simulink model "SF014A_InertiaCmpVel"  (R2013b)
settings: Solver=FixedStepDiscrete  SolverMode=SingleTasking  StartTime=0.0  StopTime=10  FixedStep=0.002  RelTol=1e-3
undefined symbols (not defined in the file): ARCHGLBPRM_2MILLISEC_SEC_F32, ARCHGLBPRM_2PI_ULS_F32, ARCHGLBPRM_PIOVER180_ULS_F32, FLTINJ_INERTIACMPVEL_INERTIACMPCMD, InertiaCmpVelDampgDecelGain, InertiaCmpVelDampgDecelGainFallSlew, InertiaCmpVelDampgGainOffThd, InertiaCmpVelDampgGainOnThd, InertiaCmpVelDecelGainEnaCal, InertiaCmpVelMotInertia, InertiaCmpVelNotchFilStruct, NOTCHFILZEROTHD_ULS_F32, SysGlbPrmSysKineRat, SysGlbPrmTorsBarStfn
libraries: FixdToFloat x13, LnrIntrpn x13, FloatToFixd x9, NxtrAbslt x4, NxtrMath x4, NxtrLim x4, simulink x2, Fil x2
(part 3 of 3)

== system SF014A_InertiaCmpVel/InertiaCmpVel/InertiaCmpVelPer1/FilterCoefCalc/Coeff_a2 ==
  FilFreqRadPs : Inport
  Constant2 : Constant  Value=ARCHGLBPRM_2MILLISEC_SEC_F32
  Constant9 : Constant  Value=2  OutDataTypeStr=single
      settings: AttributesFormatString=%<OutDataTypeStr>
  CopyRight2 : Subsystem  Description=|  mask(Copyright Information){none=on}
      | Copyright info block.                                               
      |                                                                     
      | Place copyright information at the top of every subsystem in design.
      mask prompts: none "No parameters"
      mask help: Place copyright information at the top of every subsystem in design.
      mask Display:
      | NxtrConf = 'Nexteer Confidential';
      | 
      | sys = bdroot; %handle for the current model ("system")
      | first = get_param(sys,'Created');
      | first = first(end-3:end);  %year is last four digits
      | 
      | last = get_param(sys,'LastModifiedDate');
      | if isempty(last)
      |     last = datestr(now,'yyyy');
      | else
      |     last = last(end-3:end);
      | end
      | 
      | if strcmp(first,last)
      |     fprintf('%s -- Copyright %s Nexteer',NxtrConf,first)
      | else
      |     fprintf('%s -- %s%s- %s Nexteer',NxtrConf,char(169),first,last)
      | end
  Math Function4 : Math  Operator=square  SaturateOnIntegerOverflow=on
  Product25 : Product  Inputs=**  RndMeth=Zero  OutDataTypeStr=Inherit: Same as first input
  Sum14 : Sum  OutDataTypeStr=Inherit: Same as first input
  a2 : Outport
  wires:
  FilFreqRadPs/1 -> Product25/1
  Constant2/1 -> Product25/2
  Sum14/1 -> Math Function4/1
  Math Function4/1 -> a2/1  "a2"
  Product25/1 -> Sum14/1
  Constant9/1 -> Sum14/2

== system SF014A_InertiaCmpVel/InertiaCmpVel/InertiaCmpVelPer1/FilterCoefCalc/Coeff_b0 ==
  InertiaCompCalc : Inport
  ADDCoef : Inport  Port=2
  FilFreqRadPs : Inport  Port=3
  Constant16 : Constant  Value=2  OutDataTypeStr=single
      settings: AttributesFormatString=%<OutDataTypeStr>
  Constant5 : Constant  Value=ARCHGLBPRM_2MILLISEC_SEC_F32
  Constant6 : Constant  Value=ARCHGLBPRM_2MILLISEC_SEC_F32
  CopyRight2 : Subsystem  Description=|  mask(Copyright Information){none=on}
      | Copyright info block.                                               
      |                                                                     
      | Place copyright information at the top of every subsystem in design.
      mask prompts: none "No parameters"
      mask help: Place copyright information at the top of every subsystem in design.
      mask Display:
      | NxtrConf = 'Nexteer Confidential';
      | 
      | sys = bdroot; %handle for the current model ("system")
      | first = get_param(sys,'Created');
      | first = first(end-3:end);  %year is last four digits
      | 
      | last = get_param(sys,'LastModifiedDate');
      | if isempty(last)
      |     last = datestr(now,'yyyy');
      | else
      |     last = last(end-3:end);
      | end
      | 
      | if strcmp(first,last)
      |     fprintf('%s -- Copyright %s Nexteer',NxtrConf,first)
      | else
      |     fprintf('%s -- %s%s- %s Nexteer',NxtrConf,char(169),first,last)
      | end
  Product10 : Product  Inputs=**  RndMeth=Zero  OutDataTypeStr=Inherit: Same as first input
  Product11 : Product  Inputs=**  RndMeth=Zero  OutDataTypeStr=Inherit: Same as first input
  Product23 : Product  Inputs=**  RndMeth=Zero  OutDataTypeStr=Inherit: Same as first input
  Product24 : Product  Inputs=3  RndMeth=Zero  OutDataTypeStr=Inherit: Same as first input
  Sum13 : Sum  Inputs=-+-  OutDataTypeStr=Inherit: Same as first input
  b0 : Outport
  wires:
  Constant5/1 -> Product23/1
  InertiaCompCalc/1 -> Product23/2
  Constant6/1 -> Product24/1
  FilFreqRadPs/1 -> Product24/3
  ADDCoef/1 -> Product10/1, Product24/2
  Product23/1 -> Sum13/1
  Product24/1 -> Sum13/2
  Sum13/1 -> Product11/1
  Product11/1 -> b0/1  "b0"
  Product10/1 -> Sum13/3
  Constant16/1 -> Product11/2, Product10/2

== system SF014A_InertiaCmpVel/InertiaCmpVel/InertiaCmpVelPer1/FilterCoefCalc/Coeff_b1 ==
  ADDCoef : Inport
  Constant14 : Constant  Value=2  OutDataTypeStr=single
      settings: AttributesFormatString=%<OutDataTypeStr>
  Constant17 : Constant  Value=4  OutDataTypeStr=single
      settings: AttributesFormatString=%<OutDataTypeStr>
  CopyRight2 : Subsystem  Description=|  mask(Copyright Information){none=on}
      | Copyright info block.                                               
      |                                                                     
      | Place copyright information at the top of every subsystem in design.
      mask prompts: none "No parameters"
      mask help: Place copyright information at the top of every subsystem in design.
      mask Display:
      | NxtrConf = 'Nexteer Confidential';
      | 
      | sys = bdroot; %handle for the current model ("system")
      | first = get_param(sys,'Created');
      | first = first(end-3:end);  %year is last four digits
      | 
      | last = get_param(sys,'LastModifiedDate');
      | if isempty(last)
      |     last = datestr(now,'yyyy');
      | else
      |     last = last(end-3:end);
      | end
      | 
      | if strcmp(first,last)
      |     fprintf('%s -- Copyright %s Nexteer',NxtrConf,first)
      | else
      |     fprintf('%s -- %s%s- %s Nexteer',NxtrConf,char(169),first,last)
      | end
  Product12 : Product  Inputs=**  RndMeth=Zero  OutDataTypeStr=Inherit: Same as first input
  Product8 : Product  Inputs=**  RndMeth=Zero  OutDataTypeStr=Inherit: Same as first input
  b1 : Outport
  wires:
  ADDCoef/1 -> Product8/1
  Product8/1 -> b1/1  "b1"
  Product12/1 -> Product8/2
  Constant17/1 -> Product12/1
  Constant14/1 -> Product12/2

== system SF014A_InertiaCmpVel/InertiaCmpVel/InertiaCmpVelPer1/FilterCoefCalc/Coeff_b2 ==
  InertiaCompCalc : Inport
  " FilFreqRadPs" : Inport  Port=2
  ADDCoef : Inport  Port=3
  Constant1 : Constant  Value=ARCHGLBPRM_2MILLISEC_SEC_F32
  Constant11 : Constant  Value=2  OutDataTypeStr=single
      settings: AttributesFormatString=%<OutDataTypeStr>
  Constant13 : Constant  Value=2  OutDataTypeStr=single
      settings: AttributesFormatString=%<OutDataTypeStr>
  Constant3 : Constant  Value=ARCHGLBPRM_2MILLISEC_SEC_F32
  CopyRight2 : Subsystem  Description=|  mask(Copyright Information){none=on}
      | Copyright info block.                                               
      |                                                                     
      | Place copyright information at the top of every subsystem in design.
      mask prompts: none "No parameters"
      mask help: Place copyright information at the top of every subsystem in design.
      mask Display:
      | NxtrConf = 'Nexteer Confidential';
      | 
      | sys = bdroot; %handle for the current model ("system")
      | first = get_param(sys,'Created');
      | first = first(end-3:end);  %year is last four digits
      | 
      | last = get_param(sys,'LastModifiedDate');
      | if isempty(last)
      |     last = datestr(now,'yyyy');
      | else
      |     last = last(end-3:end);
      | end
      | 
      | if strcmp(first,last)
      |     fprintf('%s -- Copyright %s Nexteer',NxtrConf,first)
      | else
      |     fprintf('%s -- %s%s- %s Nexteer',NxtrConf,char(169),first,last)
      | end
  Product21 : Product  Inputs=**  RndMeth=Zero  OutDataTypeStr=Inherit: Same as first input
  Product22 : Product  Inputs=3  RndMeth=Zero  OutDataTypeStr=Inherit: Same as first input
  Product6 : Product  Inputs=**  RndMeth=Zero  OutDataTypeStr=Inherit: Same as first input
  Product7 : Product  Inputs=**  RndMeth=Zero  OutDataTypeStr=Inherit: Same as first input
  Sum12 : Sum  Inputs=+--  OutDataTypeStr=Inherit: Same as first input
  b2 : Outport
  wires:
  Constant3/1 -> Product21/1
  InertiaCompCalc/1 -> Product21/2
  Constant1/1 -> Product22/1
  " FilFreqRadPs"/1 -> Product22/3
  ADDCoef/1 -> Product6/1, Product22/2
  Product21/1 -> Sum12/1
  Product22/1 -> Sum12/2
  Product6/1 -> Sum12/3
  Product7/1 -> b2/1  "b2"
  Constant11/1 -> Product6/2
  Sum12/1 -> Product7/1
  Constant13/1 -> Product7/2

== system SF014A_InertiaCmpVel/InertiaCmpVel/InertiaCmpVelPer1/FilterCoefCalc/CopyRight2 ==

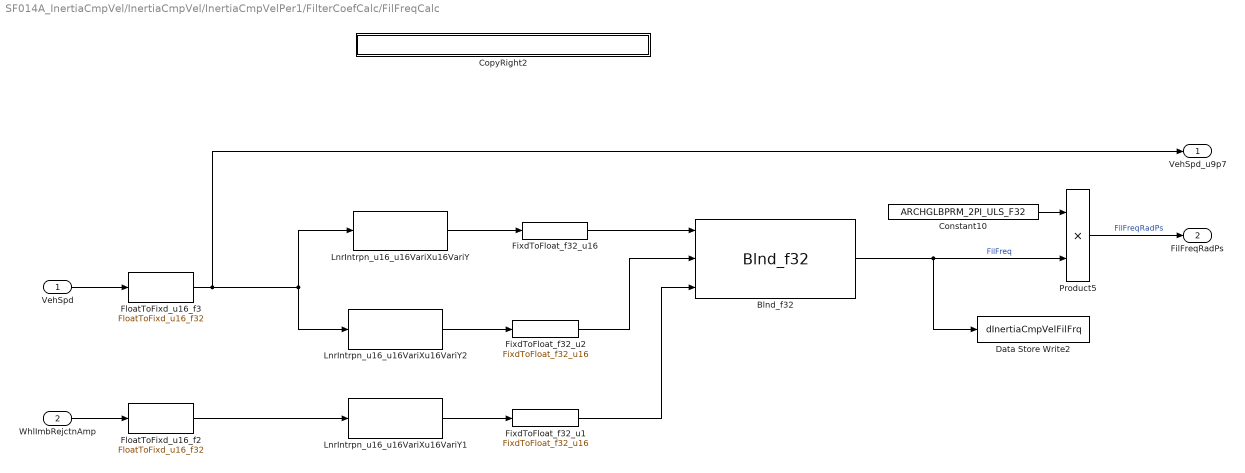
== system SF014A_InertiaCmpVel/InertiaCmpVel/InertiaCmpVelPer1/FilterCoefCalc/FilFreqCalc ==
  VehSpd : Inport
  WhlImbRejctnAmp : Inport  Port=2
  Blnd_f32 : NxtrMath/Blnd_f32  SFunctionSpec=single y1 = Blnd_f32(single u1, single u2, single u3)  Parameter3=on
      settings: AttributesFormatString=%<Name>
  Constant10 : Constant  Value=ARCHGLBPRM_2PI_ULS_F32
  CopyRight2 : Subsystem  Description=|  mask(Copyright Information){none=on}
      | Copyright info block.                                               
      |                                                                     
      | Place copyright information at the top of every subsystem in design.
      mask prompts: none "No parameters"
      mask help: Place copyright information at the top of every subsystem in design.
      mask Display:
      | NxtrConf = 'Nexteer Confidential';
      | 
      | sys = bdroot; %handle for the current model ("system")
      | first = get_param(sys,'Created');
      | first = first(end-3:end);  %year is last four digits
      | 
      | last = get_param(sys,'LastModifiedDate');
      | if isempty(last)
      |     last = datestr(now,'yyyy');
      | else
      |     last = last(end-3:end);
      | end
      | 
      | if strcmp(first,last)
      |     fprintf('%s -- Copyright %s Nexteer',NxtrConf,first)
      | else
      |     fprintf('%s -- %s%s- %s Nexteer',NxtrConf,char(169),first,last)
      | end
  Data Store Write2 : DataStoreWrite  DataStoreName=dInertiaCmpVelFilFrq
  FixdToFloat_f32_u1 : FixdToFloat/FixdToFloat_f32_u16  Param1=9
  FixdToFloat_f32_u16 : FixdToFloat/FixdToFloat_f32_u16  Param1=9
  FixdToFloat_f32_u2 : FixdToFloat/FixdToFloat_f32_u16  Param1=9
  FloatToFixd_u16_f2 : FloatToFixd/FloatToFixd_u16_f32  Param1=12
  FloatToFixd_u16_f3 : FloatToFixd/FloatToFixd_u16_f32  Param1=7
  LnrIntrpn_u16_u16VariXu16VariY : LnrIntrpn/LnrIntrpn_u16_u16VariXu16VariY  XTbl=SysGlbPrmVehSpdBilnrSeln  YTbl=InertiaCmpVelDampgFilFrq
      settings: AttributesFormatString=Lnr ( u16VariX , u16VariY )
  LnrIntrpn_u16_u16VariXu16VariY1 : LnrIntrpn/LnrIntrpn_u16_u16VariXu16VariY  XTbl=InertiaCmpVelDampgWhlImbRejctnBlndX  YTbl=InertiaCmpVelDampgWhlImbRejctnBlndY
      settings: AttributesFormatString=Lnr ( u16VariX , u16VariY )
  LnrIntrpn_u16_u16VariXu16VariY2 : LnrIntrpn/LnrIntrpn_u16_u16VariXu16VariY  XTbl=SysGlbPrmVehSpdBilnrSeln  YTbl=InertiaCmpVelDampgFilFrqWhlImbRejctnOn
      settings: AttributesFormatString=Lnr ( u16VariX , u16VariY )
  Product5 : Product  Inputs=**  RndMeth=Zero  OutDataTypeStr=Inherit: Same as first input
  VehSpd_u9p7 : Outport
  FilFreqRadPs : Outport  Port=2
  wires:
  VehSpd/1 -> FloatToFixd_u16_f3/1
  Blnd_f32/1 -> Product5/2, Data Store Write2/1  "FilFreq"
  Product5/1 -> FilFreqRadPs/1  "FilFreqRadPs"
  Constant10/1 -> Product5/1
  FloatToFixd_u16_f3/1 -> VehSpd_u9p7/1, LnrIntrpn_u16_u16VariXu16VariY/1, LnrIntrpn_u16_u16VariXu16VariY2/1
  LnrIntrpn_u16_u16VariXu16VariY/1 -> FixdToFloat_f32_u16/1
  LnrIntrpn_u16_u16VariXu16VariY1/1 -> FixdToFloat_f32_u1/1
  FloatToFixd_u16_f2/1 -> LnrIntrpn_u16_u16VariXu16VariY1/1
  FixdToFloat_f32_u1/1 -> Blnd_f32/3
  WhlImbRejctnAmp/1 -> FloatToFixd_u16_f2/1
  LnrIntrpn_u16_u16VariXu16VariY2/1 -> FixdToFloat_f32_u2/1
  FixdToFloat_f32_u16/1 -> Blnd_f32/1
  FixdToFloat_f32_u2/1 -> Blnd_f32/2

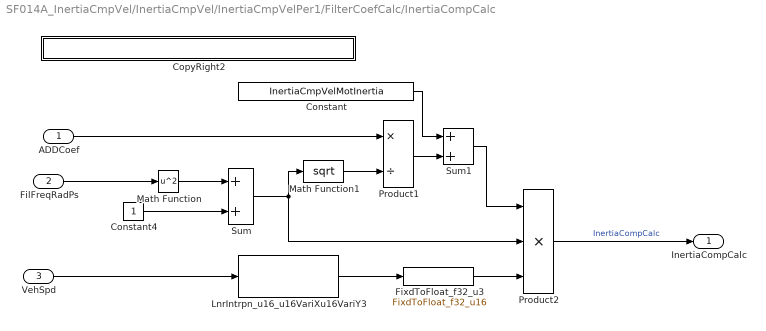
== system SF014A_InertiaCmpVel/InertiaCmpVel/InertiaCmpVelPer1/FilterCoefCalc/InertiaCompCalc ==
  ADDCoef : Inport
  FilFreqRadPs : Inport  Port=2
  VehSpd : Inport  Port=3
  Constant : Constant  Value=InertiaCmpVelMotInertia
  Constant4 : Constant  OutDataTypeStr=single
      settings: AttributesFormatString=%<OutDataTypeStr>
  CopyRight2 : Subsystem  Description=|  mask(Copyright Information){none=on}
      | Copyright info block.                                               
      |                                                                     
      | Place copyright information at the top of every subsystem in design.
      mask prompts: none "No parameters"
      mask help: Place copyright information at the top of every subsystem in design.
      mask Display:
      | NxtrConf = 'Nexteer Confidential';
      | 
      | sys = bdroot; %handle for the current model ("system")
      | first = get_param(sys,'Created');
      | first = first(end-3:end);  %year is last four digits
      | 
      | last = get_param(sys,'LastModifiedDate');
      | if isempty(last)
      |     last = datestr(now,'yyyy');
      | else
      |     last = last(end-3:end);
      | end
      | 
      | if strcmp(first,last)
      |     fprintf('%s -- Copyright %s Nexteer',NxtrConf,first)
      | else
      |     fprintf('%s -- %s%s- %s Nexteer',NxtrConf,char(169),first,last)
      | end
  FixdToFloat_f32_u3 : FixdToFloat/FixdToFloat_f32_u16  Param1=14
  LnrIntrpn_u16_u16VariXu16VariY3 : LnrIntrpn/LnrIntrpn_u16_u16VariXu16VariY  XTbl=SysGlbPrmVehSpdBilnrSeln  YTbl=InertiaCmpVelCmdScaY
      settings: AttributesFormatString=Lnr ( u16VariX , u16VariY )
  Math Function : Math  Operator=square  SaturateOnIntegerOverflow=on
  Math Function1 : Math  Operator=sqrt  SaturateOnIntegerOverflow=on
  Product1 : Product  Inputs=*/  RndMeth=Zero  OutDataTypeStr=Inherit: Same as first input
  Product2 : Product  Inputs=3  RndMeth=Zero  OutDataTypeStr=Inherit: Same as first input
  Sum : Sum  OutDataTypeStr=Inherit: Same as first input
  Sum1 : Sum  OutDataTypeStr=Inherit: Same as first input
  InertiaCompCalc : Outport
  wires:
  FilFreqRadPs/1 -> Math Function/1
  Math Function/1 -> Sum/1
  Constant4/1 -> Sum/2
  Sum/1 -> Product2/2, Math Function1/1
  ADDCoef/1 -> Product1/1
  Math Function1/1 -> Product1/2
  Constant/1 -> Sum1/1
  Product1/1 -> Sum1/2
  Sum1/1 -> Product2/1
  Product2/1 -> InertiaCompCalc/1  "InertiaCompCalc"
  LnrIntrpn_u16_u16VariXu16VariY3/1 -> FixdToFloat_f32_u3/1
  VehSpd/1 -> LnrIntrpn_u16_u16VariXu16VariY3/1
  FixdToFloat_f32_u3/1 -> Product2/3

== system SF014A_InertiaCmpVel/InertiaCmpVel/InertiaCmpVelPer1/GenFddIcCmd/CopyRight2 ==

== system SF014A_InertiaCmpVel/InertiaCmpVel/InertiaCmpVelPer1/Inertia Comp Notch Compensation/CopyRight2 ==

== system SF014A_InertiaCmpVel/InertiaCmpVel/InertiaCmpVelPer1/Inertia Comp Notch Compensation/NotchFilter ==
  InertiaComp : Inport
  CopyRight2 : Subsystem  Description=|  mask(Copyright Information){none=on}
      | Copyright info block.                                               
      |                                                                     
      | Place copyright information at the top of every subsystem in design.
      mask prompts: none "No parameters"
      mask help: Place copyright information at the top of every subsystem in design.
      mask Display:
      | NxtrConf = 'Nexteer Confidential';
      | 
      | sys = bdroot; %handle for the current model ("system")
      | first = get_param(sys,'Created');
      | first = first(end-3:end);  %year is last four digits
      | 
      | last = get_param(sys,'LastModifiedDate');
      | if isempty(last)
      |     last = datestr(now,'yyyy');
      | else
      |     last = last(end-3:end);
      | end
      | 
      | if strcmp(first,last)
      |     fprintf('%s -- Copyright %s Nexteer',NxtrConf,first)
      | else
      |     fprintf('%s -- %s%s- %s Nexteer',NxtrConf,char(169),first,last)
      | end
  Data Store Read : DataStoreRead  RequirementInfo="{'linktype_rmi_doors' '0000a52e (/E-STEER Core/SubSystem Specifications/Application Functions/SF014A Inertia Compensation)' '#SF014A_59' 'true' 'REQ:  SF014A_59' '' ; 'linktype_rmi_doors' '0000a52e (/E-STEER Core/SubSystem Specifications/Application Functions/SF014A Inertia Compensation)' '#SF014A_102' 'true' 'REQ:  SF014A_102' '' } %GIDa_dc21cdc0_c6e5_4d11_9229_19c8861a3c5e"  DataStoreName=NotchFilChk
  If : If  RequirementInfo="{'linktype_rmi_doors' '0000a52e (/E-STEER Core/SubSystem Specifications/Application Functions/SF014A Inertia Compensation)' '#SF014A_59' 'true' 'REQ:  SF014A_59' '' ; 'linktype_rmi_doors' '0000a52e (/E-STEER Core/SubSystem Specifications/Application Functions/SF014A Inertia Compensation)' '#SF014A_102' 'true' 'REQ:  SF014A_102' '' } %GIDa_70f26406_49c6_4e07_bcec_1e6c3e012c86"  IfExpression=u1
  Merge : Merge
  NotchFilterDisable : Subsystem  RequirementInfo="{'linktype_rmi_doors' '0000a52e (/E-STEER Core/SubSystem Specifications/Application Functions/SF014A Inertia Compensation)' '#SF014A_102' 'true' 'REQ:  SF014A_102' '' } %GIDa_30184175_afde_4ff1_8b23_6765ba77d169"  TreatAsAtomicUnit=on
  NotchFilterEnable : Subsystem  RequirementInfo="{'linktype_rmi_doors' '0000a52e (/E-STEER Core/SubSystem Specifications/Application Functions/SF014A Inertia Compensation)' '#SF014A_59' 'true' 'REQ:  SF014A_59' '' } %GIDa_a915e864_4481_45a3_be53_f1b7cc69e14b"  TreatAsAtomicUnit=on
  CompVelOutp : Outport
  wires:
  InertiaComp/1 -> NotchFilterDisable/1(InertiaComp), NotchFilterEnable/1(InertiaComp)
  NotchFilterEnable/1(CompVelOutp) -> Merge/1
  If/1 -> NotchFilterEnable/Action
  NotchFilterDisable/1(InertiaCompOutp) -> Merge/2
  If/2 -> NotchFilterDisable/Action
  Merge/1 -> CompVelOutp/1
  Data Store Read/1 -> If/1

== system SF014A_InertiaCmpVel/InertiaCmpVel/InertiaCmpVelPer1/InertiaCmpVelCmdDisable/CopyRight2 ==

== system SF014A_InertiaCmpVel/InertiaCmpVel/InertiaCmpVelPer1/InertiaCmpVelCmdEnable/CopyRight2 ==

== system SF014A_InertiaCmpVel/InertiaCmpVel/InertiaCmpVelPer1/ADDCoefCalc/DecelGain/CopyRight2 ==

== system SF014A_InertiaCmpVel/InertiaCmpVel/InertiaCmpVelPer1/ADDCoefCalc/DecelGain/DecelGainCalc1 ==
  Action Port : ActionPort  ActionType=then
  Constant7 : Constant  Value=InertiaCmpVelDampgDecelGain
  CopyRight2 : Subsystem  Description=|  mask(Copyright Information){none=on}
      | Copyright info block.                                               
      |                                                                     
      | Place copyright information at the top of every subsystem in design.
      mask prompts: none "No parameters"
      mask help: Place copyright information at the top of every subsystem in design.
      mask Display:
      | NxtrConf = 'Nexteer Confidential';
      | 
      | sys = bdroot; %handle for the current model ("system")
      | first = get_param(sys,'Created');
      | first = first(end-3:end);  %year is last four digits
      | 
      | last = get_param(sys,'LastModifiedDate');
      | if isempty(last)
      |     last = datestr(now,'yyyy');
      | else
      |     last = last(end-3:end);
      | end
      | 
      | if strcmp(first,last)
      |     fprintf('%s -- Copyright %s Nexteer',NxtrConf,first)
      | else
      |     fprintf('%s -- %s%s- %s Nexteer',NxtrConf,char(169),first,last)
      | end
  RawDecelGain : Outport
  wires:
  Constant7/1 -> RawDecelGain/1

== system SF014A_InertiaCmpVel/InertiaCmpVel/InertiaCmpVelPer1/ADDCoefCalc/DecelGain/DecelGainCalc2 ==
  Action Port : ActionPort  ActionType=elseif
  Constant4 : Constant  OutDataTypeStr=single
      settings: AttributesFormatString=%<OutDataTypeStr>
  CopyRight2 : Subsystem  Description=|  mask(Copyright Information){none=on}
      | Copyright info block.                                               
      |                                                                     
      | Place copyright information at the top of every subsystem in design.
      mask prompts: none "No parameters"
      mask help: Place copyright information at the top of every subsystem in design.
      mask Display:
      | NxtrConf = 'Nexteer Confidential';
      | 
      | sys = bdroot; %handle for the current model ("system")
      | first = get_param(sys,'Created');
      | first = first(end-3:end);  %year is last four digits
      | 
      | last = get_param(sys,'LastModifiedDate');
      | if isempty(last)
      |     last = datestr(now,'yyyy');
      | else
      |     last = last(end-3:end);
      | end
      | 
      | if strcmp(first,last)
      |     fprintf('%s -- Copyright %s Nexteer',NxtrConf,first)
      | else
      |     fprintf('%s -- %s%s- %s Nexteer',NxtrConf,char(169),first,last)
      | end
  RawDecelGain : Outport
  wires:
  Constant4/1 -> RawDecelGain/1

== system SF014A_InertiaCmpVel/InertiaCmpVel/InertiaCmpVelPer1/ADDCoefCalc/DecelGain/DecelGainCalc3 ==
  Action Port : ActionPort  ActionType=else
  CopyRight2 : Subsystem  Description=|  mask(Copyright Information){none=on}
      | Copyright info block.                                               
      |                                                                     
      | Place copyright information at the top of every subsystem in design.
      mask prompts: none "No parameters"
      mask help: Place copyright information at the top of every subsystem in design.
      mask Display:
      | NxtrConf = 'Nexteer Confidential';
      | 
      | sys = bdroot; %handle for the current model ("system")
      | first = get_param(sys,'Created');
      | first = first(end-3:end);  %year is last four digits
      | 
      | last = get_param(sys,'LastModifiedDate');
      | if isempty(last)
      |     last = datestr(now,'yyyy');
      | else
      |     last = last(end-3:end);
      | end
      | 
      | if strcmp(first,last)
      |     fprintf('%s -- Copyright %s Nexteer',NxtrConf,first)
      | else
      |     fprintf('%s -- %s%s- %s Nexteer',NxtrConf,char(169),first,last)
      | end
  Data Store Read : DataStoreRead  DataStoreName=DecelGain
  RawDecelGain : Outport
  wires:
  Data Store Read/1 -> RawDecelGain/1

== system SF014A_InertiaCmpVel/InertiaCmpVel/InertiaCmpVelPer1/ADDCoefCalc/DecelGainDisable/CopyRight2 ==

== system SF014A_InertiaCmpVel/InertiaCmpVel/InertiaCmpVelPer1/ADDCoefCalc/DecelGainEnable/CopyRight2 ==

== system SF014A_InertiaCmpVel/InertiaCmpVel/InertiaCmpVelPer1/FilterCoefCalc/Coeff_a0/CopyRight2 ==

== system SF014A_InertiaCmpVel/InertiaCmpVel/InertiaCmpVelPer1/FilterCoefCalc/Coeff_a1/CopyRight2 ==

== system SF014A_InertiaCmpVel/InertiaCmpVel/InertiaCmpVelPer1/FilterCoefCalc/Coeff_a2/CopyRight2 ==

== system SF014A_InertiaCmpVel/InertiaCmpVel/InertiaCmpVelPer1/FilterCoefCalc/Coeff_b0/CopyRight2 ==

== system SF014A_InertiaCmpVel/InertiaCmpVel/InertiaCmpVelPer1/FilterCoefCalc/Coeff_b1/CopyRight2 ==

== system SF014A_InertiaCmpVel/InertiaCmpVel/InertiaCmpVelPer1/FilterCoefCalc/Coeff_b2/CopyRight2 ==

== system SF014A_InertiaCmpVel/InertiaCmpVel/InertiaCmpVelPer1/FilterCoefCalc/FilFreqCalc/CopyRight2 ==

== system SF014A_InertiaCmpVel/InertiaCmpVel/InertiaCmpVelPer1/FilterCoefCalc/InertiaCompCalc/CopyRight2 ==

== system SF014A_InertiaCmpVel/InertiaCmpVel/InertiaCmpVelPer1/Inertia Comp Notch Compensation/NotchFilter/CopyRight2 ==

== system SF014A_InertiaCmpVel/InertiaCmpVel/InertiaCmpVelPer1/Inertia Comp Notch Compensation/NotchFilter/NotchFilterDisable ==
  InertiaComp : Inport
  Action Port : ActionPort  ActionType=else
  CopyRight2 : Subsystem  Description=|  mask(Copyright Information){none=on}
      | Copyright info block.                                               
      |                                                                     
      | Place copyright information at the top of every subsystem in design.
      mask prompts: none "No parameters"
      mask help: Place copyright information at the top of every subsystem in design.
      mask Display:
      | NxtrConf = 'Nexteer Confidential';
      | 
      | sys = bdroot; %handle for the current model ("system")
      | first = get_param(sys,'Created');
      | first = first(end-3:end);  %year is last four digits
      | 
      | last = get_param(sys,'LastModifiedDate');
      | if isempty(last)
      |     last = datestr(now,'yyyy');
      | else
      |     last = last(end-3:end);
      | end
      | 
      | if strcmp(first,last)
      |     fprintf('%s -- Copyright %s Nexteer',NxtrConf,first)
      | else
      |     fprintf('%s -- %s%s- %s Nexteer',NxtrConf,char(169),first,last)
      | end
  InertiaCompOutp : Outport
  wires:
  InertiaComp/1 -> InertiaCompOutp/1

== system SF014A_InertiaCmpVel/InertiaCmpVel/InertiaCmpVelPer1/Inertia Comp Notch Compensation/NotchFilter/NotchFilterEnable ==
  InertiaComp : Inport
  Action Port : ActionPort  ActionType=then
  CopyRight2 : Subsystem  Description=|  mask(Copyright Information){none=on}
      | Copyright info block.                                               
      |                                                                     
      | Place copyright information at the top of every subsystem in design.
      mask prompts: none "No parameters"
      mask help: Place copyright information at the top of every subsystem in design.
      mask Display:
      | NxtrConf = 'Nexteer Confidential';
      | 
      | sys = bdroot; %handle for the current model ("system")
      | first = get_param(sys,'Created');
      | first = first(end-3:end);  %year is last four digits
      | 
      | last = get_param(sys,'LastModifiedDate');
      | if isempty(last)
      |     last = datestr(now,'yyyy');
      | else
      |     last = last(end-3:end);
      | end
      | 
      | if strcmp(first,last)
      |     fprintf('%s -- Copyright %s Nexteer',NxtrConf,first)
      | else
      |     fprintf('%s -- %s%s- %s Nexteer',NxtrConf,char(169),first,last)
      | end
  InertiaCompNotch : Subsystem  mask(FilNotchFullUpdOutp_f32){StVarGain=InertiaCmpVelNotchFilStruct, StVarSt=TqSnsrVelFilNotchSt}
      mask prompts: StVarGain "State Variable For Gain"; StVarSt "State Variable For State"
      mask help: It Calculates notch filter output and state information for next sample
      mask init:
      | blk = gcb;
      | set_param([ blk '/Data Store Read'],'DataStoreName',StVarSt)
      | set_param([ blk '/Data Store Read1'],'DataStoreName',StVarSt)
      | set_param([ blk '/Data Store Write'],'DataStoreName',StVarSt)
      | set_param([ blk '/Data Store Write1'],'DataStoreName',StVarSt)
      | set_param([ blk '/CompFilter_FwdPath/Constant'],'Value',[StVarGain '.FilGainB0'])
      | set_param([ blk '/CompFilter_UpdateSV/Constant'],'Value',[StVarGain '.FilGainB1'])
      | set_param([ blk '/CompFilter_UpdateSV/Constant1'],'Value',[StVarGain '.FilGainA1'])
      | set_param([ blk '/CompFilter_UpdateSV/Constant2'],'Value',[StVarGain '.FilGainB2'])
      | set_param([ blk '/CompFilter_UpdateSV/Constant3'],'Value',[StVarGain '.FilGainA2'])
      | 
      | 
      | 
      | try
      |     dt1 = evalin('base',[StVarSt '.EngDT']);
      | catch err
      |     if strcmp(err.identifier,'MATLAB:undefinedVarOrClass')
      |         dt1 = struct.FilNotchStRec1;
      |     end
      | end
      | 
      | 
      | if isa(dt1,'struct.FilNotchStRec1')
      |     set_param([ blk '/Data Store Read'],'DataStoreElements',[StVarSt '.FilSt1'])
      |     set_param([ blk '/Data Store Read1'],'DataStoreElements',[StVarSt '.FilSt2'])
      |     set_param([ blk '/Data Store Write'],'DataStoreElements',[StVarSt '.FilSt1'])
      |     set_param([ blk '/Data Store Write1'],'DataStoreElements',[StVarSt '.FilSt2'])
      |     
      | else
      |     error('Incorrect data class.');
      | end
      settings: AttributesFormatString=%<Tag>
      mask Display:
      | text(0.35,0.9,'FilNotchUpd')
      | 
      | port_label('input',1,'Inp')
      | port_label('output',1,'Outp')
  CompVelOutp : Outport
  wires:
  InertiaCompNotch/1(Comp_vel_Output) -> CompVelOutp/1
  InertiaComp/1 -> InertiaCompNotch/1(InertiaComp)

== system SF014A_InertiaCmpVel/InertiaCmpVel/InertiaCmpVelPer1/ADDCoefCalc/DecelGain/DecelGainCalc1/CopyRight2 ==

== system SF014A_InertiaCmpVel/InertiaCmpVel/InertiaCmpVelPer1/ADDCoefCalc/DecelGain/DecelGainCalc2/CopyRight2 ==

== system SF014A_InertiaCmpVel/InertiaCmpVel/InertiaCmpVelPer1/ADDCoefCalc/DecelGain/DecelGainCalc3/CopyRight2 ==

== system SF014A_InertiaCmpVel/InertiaCmpVel/InertiaCmpVelPer1/Inertia Comp Notch Compensation/NotchFilter/NotchFilterDisable/CopyRight2 ==

== system SF014A_InertiaCmpVel/InertiaCmpVel/InertiaCmpVelPer1/Inertia Comp Notch Compensation/NotchFilter/NotchFilterEnable/CopyRight2 ==

== system SF014A_InertiaCmpVel/InertiaCmpVel/InertiaCmpVelPer1/Inertia Comp Notch Compensation/NotchFilter/NotchFilterEnable/InertiaCompNotch ==
  InertiaComp : Inport
  CompFilter_FwdPath : Subsystem
  CompFilter_UpdateSV : Subsystem
  Data Store Read : DataStoreRead  Priority=1  DataStoreName=TqSnsrVelFilNotchSt  DataStoreElements=TqSnsrVelFilNotchSt.FilSt1
      settings: AttributesFormatString=Priority:%<Priority>
  Data Store Read1 : DataStoreRead  Priority=1  DataStoreName=TqSnsrVelFilNotchSt  DataStoreElements=TqSnsrVelFilNotchSt.FilSt2
      settings: AttributesFormatString=Priority:%<Priority>
  Data Store Write : DataStoreWrite  Priority=2  DataStoreName=TqSnsrVelFilNotchSt  DataStoreElements=TqSnsrVelFilNotchSt.FilSt1
      settings: AttributesFormatString=Priority:%<Priority>
  Data Store Write1 : DataStoreWrite  Priority=2  DataStoreName=TqSnsrVelFilNotchSt  DataStoreElements=TqSnsrVelFilNotchSt.FilSt2
      settings: AttributesFormatString=Priority:%<Priority>
  Comp_vel_Output : Outport
  wires:
  InertiaComp/1 -> CompFilter_FwdPath/1(Inertiacomp), CompFilter_UpdateSV/1(Inertia_comp)
  CompFilter_FwdPath/1(CompFilterOut) -> Comp_vel_Output/1, CompFilter_UpdateSV/2(CompFiltOut)
  CompFilter_UpdateSV/1(CompFiltSV1) -> Data Store Write/1
  Data Store Read/1 -> CompFilter_FwdPath/2(PrevCompFiltSV1)
  CompFilter_UpdateSV/2(CompFiltSV2) -> Data Store Write1/1
  Data Store Read1/1 -> CompFilter_UpdateSV/3(PrevCompFiltSV2)

== system SF014A_InertiaCmpVel/InertiaCmpVel/InertiaCmpVelPer1/Inertia Comp Notch Compensation/NotchFilter/NotchFilterEnable/InertiaCompNotch/CompFilter_FwdPath ==
  Inertiacomp : Inport
  PrevCompFiltSV1 : Inport  Port=2
  Constant : Constant  Value=InertiaCmpVelNotchFilStruct.FilGainB0
  Product : Product
  Sum3 : Sum  Inputs=|++  OutDataTypeStr=single  RndMeth=Zero
  CompFilterOut : Outport
  wires:
  Sum3/1 -> CompFilterOut/1
  Product/1 -> Sum3/1
  PrevCompFiltSV1/1 -> Sum3/2
  Inertiacomp/1 -> Product/1
  Constant/1 -> Product/2

== system SF014A_InertiaCmpVel/InertiaCmpVel/InertiaCmpVelPer1/Inertia Comp Notch Compensation/NotchFilter/NotchFilterEnable/InertiaCompNotch/CompFilter_UpdateSV ==
  Inertia_comp : Inport
  CompFiltOut : Inport  Port=2
  PrevCompFiltSV2 : Inport  Port=3
  Constant : Constant  Value=InertiaCmpVelNotchFilStruct.FilGainB1
  Constant1 : Constant  Value=InertiaCmpVelNotchFilStruct.FilGainA1
  Constant2 : Constant  Value=InertiaCmpVelNotchFilStruct.FilGainB2
  Constant3 : Constant  Value=InertiaCmpVelNotchFilStruct.FilGainA2
  Product{,1..3} (4 alike) : Product
  Sum : Sum  Inputs=|+-  OutDataTypeStr=single  RndMeth=Zero
  Sum1 : Sum  Inputs=++-  OutDataTypeStr=single  RndMeth=Zero
  CompFiltSV1 : Outport
  CompFiltSV2 : Outport  Port=2
  wires:
  Inertia_comp/1 -> Product/1, Product1/1
  Product1/1 -> Sum/1
  Sum/1 -> CompFiltSV2/1
  PrevCompFiltSV2/1 -> Sum1/1
  Sum1/1 -> CompFiltSV1/1
  Product3/1 -> Sum/2
  Product2/1 -> Sum1/3
  CompFiltOut/1 -> Product3/1, Product2/2
  Constant/1 -> Product/2
  Constant2/1 -> Product1/2
  Product/1 -> Sum1/2
  Constant3/1 -> Product3/2
  Constant1/1 -> Product2/1
